simulink subsystem "April_Tag_Errors"  (R2023b)
settings: Solver=VariableStepAuto  StartTime=0.0  StopTime=10.0  RelTol=1e-3
undefined symbols (not defined in the file): AT_Reef_Target_Center_X, AT_Reef_Target_Center_Y, AT_Reef_Target_Left_Y, AT_Reef_Target_Poles_X, AT_Reef_Target_Right_Y
libraries: simulink x3
settings Model: Creator=ander  LastModifiedBy=ander

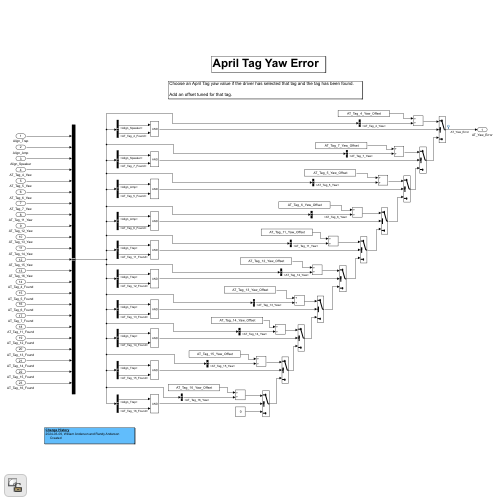
[thumbnail: Simulink's stored preview of the top-level diagram]
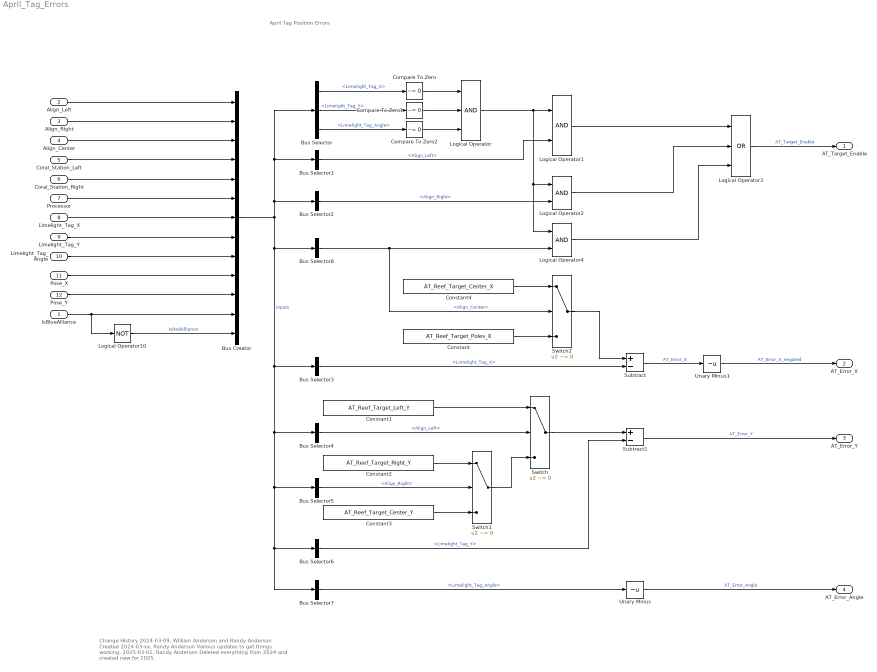
== system April_Tag_Errors ==
  note: Change History
      | 2024-03-09, William Anderson and Randy Anderson
      | Created
      | 2024-03-xx, Randy Anderson
      | Various updates to get things working.
      | 2025-03-01, Randy Anderosn
      | Deleted everything from 2024 and created new for 2025.
  note: April Tag Position Errors
  IsBlueAlliance : Inport
  Align_Left : Inport  Port=2
  Align_Right : Inport  Port=3
  Align_Center : Inport  Port=4
  Coral_Station_Left : Inport  Port=5
  Coral_Station_Right : Inport  Port=6
  Processor : Inport  Port=7
  Limelight_Tag_X : Inport  Port=8
  Limelight_Tag_Y : Inport  Port=9
  Limelight_Tag_Angle : Inport  Port=10
  Pose_X : Inport  Port=11
  Pose_Y : Inport  Port=12
  Bus Creator : BusCreator  Inputs=13
  Bus Selector : BusSelector  OutputSignals=Limelight_Tag_X,Limelight_Tag_Y,Limelight_Tag_Angle
  Bus Selector1 : BusSelector  OutputSignals=Align_Left
  Bus Selector2 : BusSelector  OutputSignals=Align_Right
  Bus Selector3 : BusSelector  OutputSignals=Limelight_Tag_X
  Bus Selector4 : BusSelector  OutputSignals=Align_Left
  Bus Selector5 : BusSelector  OutputSignals=Align_Right
  Bus Selector6 : BusSelector  OutputSignals=Limelight_Tag_Y
  Bus Selector7 : BusSelector  OutputSignals=Limelight_Tag_Angle
  Bus Selector8 : BusSelector  OutputSignals=Align_Center
  Compare To Zero : simulink/Logic and Bit Operations/Compare To Zero  relop=~=  OutDataTypeStr=boolean
  Compare To Zero1 : simulink/Logic and Bit Operations/Compare To Zero  relop=~=  OutDataTypeStr=boolean
  Compare To Zero2 : simulink/Logic and Bit Operations/Compare To Zero  relop=~=  OutDataTypeStr=boolean
  Constant : Constant  Value=AT_Reef_Target_Poles_X
  Constant1 : Constant  Value=AT_Reef_Target_Left_Y
  Constant2 : Constant  Value=AT_Reef_Target_Right_Y
  Constant3 : Constant  Value=AT_Reef_Target_Center_Y
  Constant4 : Constant  Value=AT_Reef_Target_Center_X
  Logical Operator : Logic  Inputs=3  AllPortsSameDT=off  OutDataTypeStr=boolean
  Logical Operator1 : Logic  AllPortsSameDT=off  OutDataTypeStr=boolean
  Logical Operator10 : Logic  Operator=NOT  AllPortsSameDT=off  OutDataTypeStr=boolean
  Logical Operator2 : Logic  AllPortsSameDT=off  OutDataTypeStr=boolean
  Logical Operator3 : Logic  Operator=OR  Inputs=3  AllPortsSameDT=off  OutDataTypeStr=boolean
  Logical Operator4 : Logic  AllPortsSameDT=off  OutDataTypeStr=boolean
  Subtract : Sum  Inputs=+-
  Subtract1 : Sum  Inputs=+-
  Switch : Switch  Criteria=u2 ~= 0  SaturateOnIntegerOverflow=off  InputSameDT=off
  Switch1 : Switch  Criteria=u2 ~= 0  SaturateOnIntegerOverflow=off  InputSameDT=off
  Switch2 : Switch  Criteria=u2 ~= 0  SaturateOnIntegerOverflow=off  InputSameDT=off
  Unary Minus : UnaryMinus
  Unary Minus1 : UnaryMinus
  AT_Target_Enable : Outport
  AT_Error_X : Outport  Port=2
  AT_Error_Y : Outport  Port=3
  AT_Error_Angle : Outport  Port=4
  wires:
  Logical Operator10/1 -> Bus Creator/13  "IsRedAlliance"
  IsBlueAlliance/1 -> Bus Creator/12, Logical Operator10/1
  Pose_Y/1 -> Bus Creator/11
  Pose_X/1 -> Bus Creator/10
  Limelight_Tag_Angle/1 -> Bus Creator/9
  Limelight_Tag_Y/1 -> Bus Creator/8
  Limelight_Tag_X/1 -> Bus Creator/7
  Align_Right/1 -> Bus Creator/2
  Align_Left/1 -> Bus Creator/1
  Align_Center/1 -> Bus Creator/3
  Bus Creator/1 -> Bus Selector/1, Bus Selector1/1, Bus Selector2/1, Bus Selector8/1, Bus Selector3/1, Bus Selector4/1, Bus Selector6/1, Bus Selector7/1, Bus Selector5/1  "Inputs"
  Bus Selector/1 -> Compare To Zero/1  "<Limelight_Tag_X>"
  Bus Selector/2 -> Compare To Zero1/1  "<Limelight_Tag_Y>"
  Bus Selector/3 -> Compare To Zero2/1  "<Limelight_Tag_Angle>"
  Compare To Zero/1 -> Logical Operator/1
  Compare To Zero1/1 -> Logical Operator/2
  Compare To Zero2/1 -> Logical Operator/3
  Bus Selector1/1 -> Logical Operator1/2  "<Align_Left>"
  Logical Operator/1 -> Logical Operator1/1, Logical Operator4/1, Logical Operator2/1
  Bus Selector2/1 -> Logical Operator2/2  "<Align_Right>"
  Logical Operator1/1 -> Logical Operator3/1
  Logical Operator2/1 -> Logical Operator3/2
  Logical Operator3/1 -> AT_Target_Enable/1  "AT_Target_Enable"
  Bus Selector3/1 -> Subtract/2  "<Limelight_Tag_X>"
  Constant1/1 -> Switch/1
  Bus Selector4/1 -> Switch/2  "<Align_Left>"
  Switch1/1 -> Switch/3
  Bus Selector5/1 -> Switch1/2  "<Align_Right>"
  Constant2/1 -> Switch1/1
  Constant3/1 -> Switch1/3
  Switch/1 -> Subtract1/1
  Bus Selector6/1 -> Subtract1/2  "<Limelight_Tag_Y>"
  Subtract/1 -> Unary Minus1/1  "AT_Error_X"
  Subtract1/1 -> AT_Error_Y/1  "AT_Error_Y"
  Bus Selector7/1 -> Unary Minus/1  "<Limelight_Tag_Angle>"
  Unary Minus/1 -> AT_Error_Angle/1  "AT_Error_Angle"
  Unary Minus1/1 -> AT_Error_X/1  "AT_Error_X_negated"
  Bus Selector8/1 -> Logical Operator4/2, Switch2/2  "<Align_Center>"
  Logical Operator4/1 -> Logical Operator3/3
  Constant/1 -> Switch2/3
  Constant4/1 -> Switch2/1
  Switch2/1 -> Subtract/1
  Coral_Station_Left/1 -> Bus Creator/4
  Coral_Station_Right/1 -> Bus Creator/5
  Processor/1 -> Bus Creator/6
